simulink model "sfcndemo_sfun_simstate"  (Simulink 7.6)
settings: Solver=VariableStepDiscrete  StartTime=0.0  StopTime=100  MaxStep=0.001  RelTol=1e-3
settings Model: Creator=The MathWorks Inc.
settings DataIOCC: FinalStateName=finalSimState  SaveFinalState=on  SaveCompleteFinalSimState=on  SaveOutput=off  SignalLogging=off  SaveTime=off
settings OptimizationCC: InlineParams=on  EfficientMapNaN2IntZero=off
settings DebuggingCC: SolverPrmCheckMsg=error

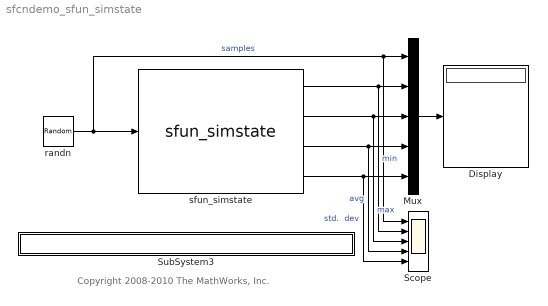
== system sfcndemo_sfun_simstate ==
  note: Copyright 2008-2010 The MathWorks, Inc.
  Display : Display
  Mux : Mux  Inputs=5
  Scope : Scope  NumInputPorts=5
      settings: TimeRange=100  YMin=-5~-5~6~2~0  YMax=10~10~10~8~3
  SubSystem3 : Subsystem  mask{filename=sfun_simstate.c}
      mask init:
      | x=sfundemo_maskdisp;
      settings: AttributesFormatString=\n  OpenFcn=sfundemo_openfcn
      mask Display: disp(x);
  randn : RandomNumber  Mean=3  Variance=9  SampleTime=1
  sfun_simstate : S-Function  FunctionName=sfun_simstate  Parameters=SimSnapCompliance, strcmp(SimStateVisibility,'on')  EnableBusSupport=off  mask(sfun_simstate){SimSnapCompliance=Custom, SimStateVisibility=off}
      mask prompts: SimSnapCompliance "Simulation Snapshot Compliance:"; SimStateVisibility "SimState visble to users"
      mask help: An Example S-Function that demonstrates the API for specifying and customizing the S-Function's Simulation State
      mask StyleString: popup(Unknown|Default|HasNoSimState|Custom|Disallow),checkbox
      mask Display:
      | fprintf('%s\n%s\n%s\n%s\n%s', ...
      |     'Demo of the API', ...
      |     'to save and restore the', ...
      |     'Simulation State of a', ...
      |     'C-Mex S-Function');
      | port_label('output', 1, 'min')
      | port_label('output', 2, 'max')
      | port_label('output', 3, 'avg')
      | port_label('output', 4, 'std')
  wires:
  randn/1 -> sfun_simstate/1, Mux/1, Scope/1  "samples"
  sfun_simstate/1 -> Mux/2, Scope/2  "min"
  sfun_simstate/2 -> Mux/3, Scope/3  "max"
  sfun_simstate/3 -> Mux/4, Scope/4  "avg"
  sfun_simstate/4 -> Mux/5, Scope/5  "std.  dev"
  Mux/1 -> Display/1

== system sfcndemo_sfun_simstate/SubSystem3 ==
